simulink model "ILC"  (R2015a)
settings: Solver=ode45  StartTime=0.0  StopTime=7  RelTol=1e-3
undefined symbols (not defined in the file or in its folder): sample_time
libraries: dspadpt3 x7
settings Model: CovSFcnEnable=off  Creator=paulghanem  LastModifiedBy=User
settings DebuggingCC: SolverPrmCheckMsg=warning

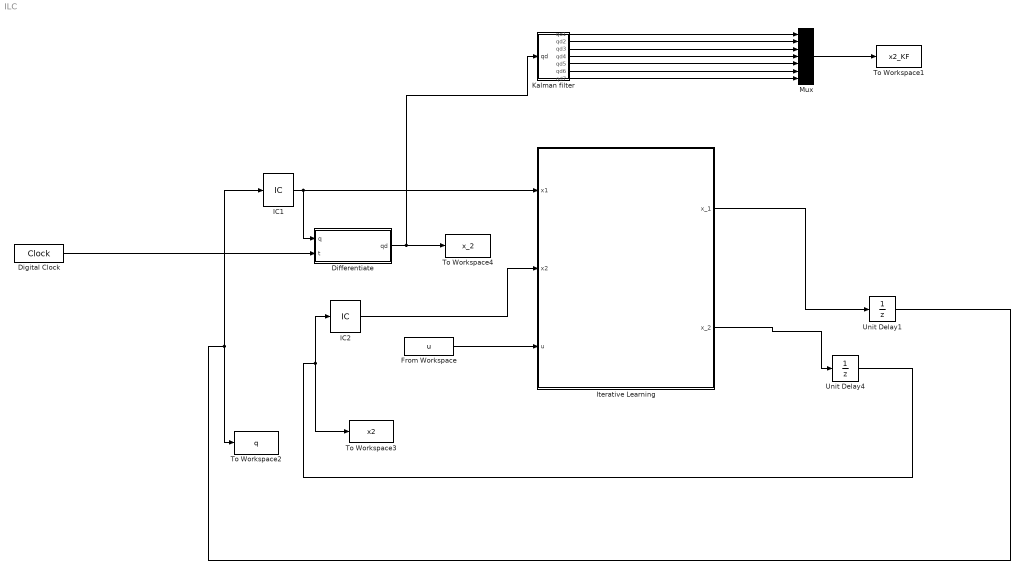
== system ILC ==
  Differentiate : Subsystem
  Digital Clock : DigitalClock  SampleTime=sample_time
  From Workspace : FromWorkspace  VariableName=u  SampleTime=sample_time
  IC1 : InitialCondition  Value=[-0.11060;-2;-0.19200;3.1;0.28250;0.09690;-0.27980]
  IC2 : InitialCondition  Value=[0 0 0 0 0 0 0]
  "Iterative Learning " : MATLAB Function  TreatAsAtomicUnit=on
  Kalman filter : Subsystem
  Mux : Mux  Inputs=7
  To Workspace1 : ToWorkspace  VariableName=x2_KF  SaveFormat=Structure With Time  SampleTime=-1
  To Workspace2 : ToWorkspace  VariableName=q  SaveFormat=Structure With Time  SampleTime=-1
  To Workspace3 : ToWorkspace  VariableName=x2  SaveFormat=Structure With Time  SampleTime=-1
  To Workspace4 : ToWorkspace  VariableName=x_2  SaveFormat=Structure With Time  SampleTime=-1
  Unit Delay1 : UnitDelay  SampleTime=sample_time
  Unit Delay4 : UnitDelay  SampleTime=sample_time
  wires:
  IC1/1 -> "Iterative Learning "/1(x1), Differentiate/1(q)
  "Iterative Learning "/1(x_1) -> Unit Delay1/1
  Unit Delay4/1 -> To Workspace3/1, IC2/1
  Unit Delay1/1 -> To Workspace2/1, IC1/1
  Digital Clock/1 -> Differentiate/2(t)
  From Workspace/1 -> "Iterative Learning "/3(u)
  IC2/1 -> "Iterative Learning "/2(x2)
  "Iterative Learning "/2(x_2) -> Unit Delay4/1
  Differentiate/1(qd) -> Kalman filter/1(qd), To Workspace4/1
  Kalman filter/1(qd1) -> Mux/1
  Kalman filter/2(qd2) -> Mux/2
  Kalman filter/3(qd3) -> Mux/3
  Kalman filter/4(qd4) -> Mux/4
  Kalman filter/5(qd5) -> Mux/5
  Kalman filter/6(qd6) -> Mux/6
  Kalman filter/7(qd7) -> Mux/7
  Mux/1 -> To Workspace1/1

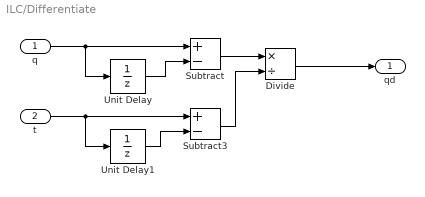
== system ILC/Differentiate ==
  q : Inport
  t : Inport  Port=2
  Divide : Product  Inputs=*/
  Subtract : Sum  Inputs=+-
  Subtract3 : Sum  Inputs=+-
  Unit Delay : UnitDelay  SampleTime=-1
  Unit Delay1 : UnitDelay  SampleTime=-1
  qd : Outport
  wires:
  q/1 -> Subtract/1, Unit Delay/1
  t/1 -> Unit Delay1/1, Subtract3/1
  Unit Delay1/1 -> Subtract3/2
  Unit Delay/1 -> Subtract/2
  Subtract/1 -> Divide/1
  Divide/1 -> qd/1
  Subtract3/1 -> Divide/2

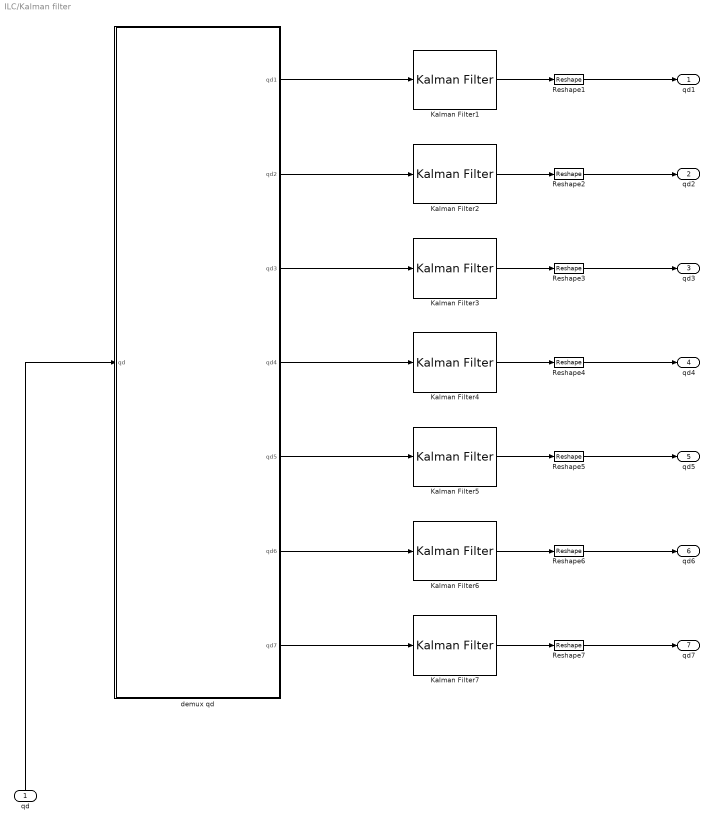
== system ILC/Kalman filter ==
  qd : Inport
  Kalman Filter1 : dspadpt3/Kalman Filter  num_targets=1  sourceEnable=Always  isReset=off  X=[-0.1106; 0]  P=[1e-4 0 ; 0 1]  A=[1 0.002 ; 0 1]  sourceMeasure=Specify via Dialog  H=[1 0]  Q=[0 0.000 ;0.000 0.004]  R=1e-3  isOutputEstMeasure=on  isOutputEstState=off  isOutputEstError=off  isOutputPrdMeasure=off  isOutputPrdState=off  isOutputPrdError=off
  Kalman Filter2 : dspadpt3/Kalman Filter  num_targets=1  sourceEnable=Always  isReset=on  X=[-1.94900000000000; 0]  P=[1e-4 0 ; 0 1]  A=[1 0.002 ; 0 1]  sourceMeasure=Specify via Dialog  H=[1 0]  Q=[0 0; 0 0.004]  R=5e-2  isOutputEstMeasure=on  isOutputEstState=off  isOutputEstError=off  isOutputPrdMeasure=off  isOutputPrdState=off  isOutputPrdError=off
  Kalman Filter3 : dspadpt3/Kalman Filter  num_targets=1  sourceEnable=Always  isReset=on  X=[-0.192000000000000; 0]  P=[1e-4 0 ; 0 1]  A=[1 0.002 ; 0 1]  sourceMeasure=Specify via Dialog  H=[1 0]  Q=[0 0; 0 0.004]  R=1e-3  isOutputEstMeasure=on  isOutputEstState=off  isOutputEstError=off  isOutputPrdMeasure=off  isOutputPrdState=off  isOutputPrdError=off
  Kalman Filter4 : dspadpt3/Kalman Filter  num_targets=1  sourceEnable=Always  isReset=on  X=[3.18400000000000; 0]  P=[1e-4 0 ; 0 1]  A=[1 0.002 ; 0 1]  sourceMeasure=Specify via Dialog  H=[1 0]  Q=[0 0; 0 0.004]  R=1e-3  isOutputEstMeasure=on  isOutputEstState=off  isOutputEstError=off  isOutputPrdMeasure=off  isOutputPrdState=off  isOutputPrdError=off
  Kalman Filter5 : dspadpt3/Kalman Filter  num_targets=1  sourceEnable=Always  isReset=on  X=[0.282500000000000; 0]  P=[1e-4 0 ; 0 1]  A=[1 0.002 ; 0 1]  sourceMeasure=Specify via Dialog  H=[1 0]  Q=[0 0; 0 0.004]  R=1e-6  isOutputEstMeasure=on  isOutputEstState=off  isOutputEstError=off  isOutputPrdMeasure=off  isOutputPrdState=off  isOutputPrdError=off
  Kalman Filter6 : dspadpt3/Kalman Filter  num_targets=1  sourceEnable=Always  isReset=on  X=[0.0969000000000000; 0]  P=[1e-4 0 ; 0 1]  A=[1 0.002 ; 0 1]  sourceMeasure=Specify via Dialog  H=[1 0]  Q=[0 0; 0 0.004]  R=1e-6  isOutputEstMeasure=on  isOutputEstState=off  isOutputEstError=off  isOutputPrdMeasure=off  isOutputPrdState=off  isOutputPrdError=off
  Kalman Filter7 : dspadpt3/Kalman Filter  num_targets=1  sourceEnable=Always  isReset=on  X=[-0.279800000000000; 0]  P=[1e-4 0 ; 0 1]  A=[1 0.002 ; 0 1]  sourceMeasure=Specify via Dialog  H=[1 0]  Q=[0 0; 0 0.004]  R=1e-6  isOutputEstMeasure=on  isOutputEstState=off  isOutputEstError=off  isOutputPrdMeasure=off  isOutputPrdState=off  isOutputPrdError=off
  Reshape{1..7} (7 alike) : Reshape
  demux qd : Subsystem
  qd1 : Outport
  qd2 : Outport  Port=2
  qd3 : Outport  Port=3
  qd4 : Outport  Port=4
  qd5 : Outport  Port=5
  qd6 : Outport  Port=6
  qd7 : Outport  Port=7
  wires:
  Reshape7/1 -> qd7/1
  Kalman Filter7/1 -> Reshape7/1
  qd/1 -> demux qd/1(qd)
  demux qd/7(qd7) -> Kalman Filter7/1
  demux qd/4(qd4) -> Kalman Filter4/1
  Kalman Filter5/1 -> Reshape5/1
  Reshape5/1 -> qd5/1
  demux qd/5(qd5) -> Kalman Filter5/1
  demux qd/2(qd2) -> Kalman Filter2/1
  demux qd/3(qd3) -> Kalman Filter3/1
  Kalman Filter3/1 -> Reshape3/1
  Kalman Filter2/1 -> Reshape2/1
  Reshape3/1 -> qd3/1
  Reshape2/1 -> qd2/1
  demux qd/6(qd6) -> Kalman Filter6/1
  Reshape6/1 -> qd6/1
  Kalman Filter6/1 -> Reshape6/1
  Kalman Filter4/1 -> Reshape4/1
  Reshape4/1 -> qd4/1
  Reshape1/1 -> qd1/1
  Kalman Filter1/1 -> Reshape1/1
  demux qd/1(qd1) -> Kalman Filter1/1

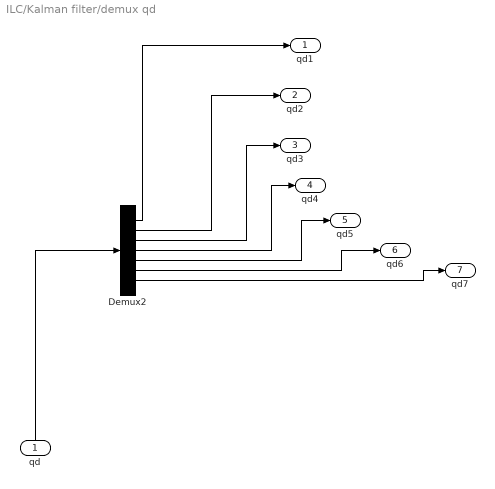
== system ILC/Kalman filter/demux qd ==
  qd : Inport
  Demux2 : Demux  Outputs=7
  qd1 : Outport
  qd2 : Outport  Port=2
  qd3 : Outport  Port=3
  qd4 : Outport  Port=4
  qd5 : Outport  Port=5
  qd6 : Outport  Port=6
  qd7 : Outport  Port=7
  wires:
  qd/1 -> Demux2/1
  Demux2/1 -> qd1/1
  Demux2/2 -> qd2/1
  Demux2/3 -> qd3/1
  Demux2/4 -> qd4/1
  Demux2/5 -> qd5/1
  Demux2/6 -> qd6/1
  Demux2/7 -> qd7/1

== matlab function ILC/Iterative Learning  ==
  data: x1 input; x2 input; u input; x_1 output; x_2 output
function [x_1,x_2]  = fcn(x1,x2,u)
%#codegen
Ts=0.002;
sig = 1e-3;

F1 =  diag([0.20519,0.094428,0.094428,0.03,0.001,0.001,0.0003]);

   C= [zeros(7,7),eye(7)];
 
 
 x11 = x1 + sig*(0.5 - rand(7,1));
 
 
 
 
 



   
    
    
    ff = G(x11);   
    
    
    
    %not to be used in real time
    U=u+ff;
    
    x_1 =  x2*Ts + x11;
    x_2 = (-inv(D(x1)+F1)*(G(x1) + bq(x2)) + inv(D(x1)+F1)*U)*Ts + x2;
     B= [zeros(7,7);inv(D(x1)+F1)];
     x_2(5:7)=zeros(3,1);
     
     
    
end 
function G=G(q)


DH_a = [0 0 0.045 -0.045 0 0 0];
    DH_d = [0 0 .55 0 0.45 0 0.061];
    DH_alpha = [-pi/2 pi/2 -pi/2 pi/2 -pi/2 pi/2 0];

    m = [10.7676 3.87 1.8022 2.4 0.1237 0.4979886 0.07548270];
    
     
    com= zeros(3,7);
    
   com(:,1) = [-0.00443422;0.12189039;-0.00066489];
    com(:,2) = [-0.00236983;0.03105614;0.01542114 ];
    com(:,3) = [-0.03825858;0.20750770;0.00003309];
    com(:,4) = [0.00498512;-0.00022942;0.13271662 ];
    com(:,5) = [0.00008921;0.00511217;0.00435824];
    com(:,6) = [-0.00012262;-0.01703194;0.02468336];
    com(:,7) = [-0.00007974;0.00016313;-0.00323552 ];
     
     % hand_mass =1.385;
      %  DH_d(7) =DH_d(7)+ .0953; % Adding the distance to the hand frame for the Schunk Gripper
       % com(:,7) =(com(:,7).*hand_mass+com(:,7).*m(7))/(hand_mass+m(7)); % Finding the combined center of mass
        %m(7) =m(7)+hand_mass;  
        
    I=zeros(3,3,7);
    T=zeros(4,4,7);
     I(:,:,1) = [0.29486350,-0.00795023,-0.00009311;
                 -0.00795023,0.11350017,-0.00018711;
                -0.00009311,-0.00018711,0.25065343];
    I(:,:,2) =[0.02606840,-0.00001346,-0.00011701;
               -0.00001346,0.01472202,0.00003659;
              -0.00011701,0.00003659,0.01934814];
    I(:,:,3) = [0.13671601,-0.01680434, 0.00000510;
               -0.01680434,0.00588354,-0.00000530;
                0.00000510,-0.00000530,0.13951371];
    I(:,:,4) = [ 0.05719268,0.00001467,0.00008193;
                 0.00001467,0.05716470,-0.00009417;
                 0.00008193,-0.00009417,0.00300441] ;
    I(:,:,5) =[0.00005587,0.00000026,.00000000;
               0.00000026,0.00007817,-0.00000083;
               0.00000000,-0.00000083,0.00006594];
    I(:,:,6) = [0.00093106,0.00000148,-0.00000201;
                0.00000148, 0.00049833,-0.00022162;
               -0.00000201,-0.00022162,0.00057483];
    I(:,:,7) = [0.003167342, 0,0;       % Approximate Inertia Tensor for Schunk Gripper
                0,0.001128942,0;
                 0,0,0.00258007;];  
            
             
for j=1:7,
        a = DH_a(j);
        d = DH_d(j);
        alpha = DH_alpha(j);
        T(:,:,j) = getTransformDH(a, d, alpha, q(j));
end 


comstar=zeros(4,7);

   
    comstar(:,1) = [com(:,1);1];
    comstar(:,2) = [com(:,2);1];
    comstar(:,3) = [com(:,3);1];
    comstar(:,4) = [com(:,4);1];
    comstar(:,5) = [com(:,5);1];
    comstar(:,6) = [com(:,6);1];
    comstar(:,7) = [com(:,7);1];
    
    Q=zeros(4,4);
    
    Q=[0,-1,0,0;
     1,0,0,0;
     0,0,0,0;
     0,0,0,0];
   
 gravity=[0,0,-9.81,0];
 G=zeros(7,1);
   G(1)= -m(1)*gravity*Q*T(:,:,1)*comstar(:,1)-m(2)*gravity*Q*T(:,:,1)*T(:,:,2)*comstar(:,2)-m(3)*gravity*Q*T(:,:,1)*T(:,:,2)*T(:,:,3)*comstar(:,3)-m(4)*gravity*Q*T(:,:,1)*T(:,:,2)*T(:,:,3)*T(:,:,4)*comstar(:,4)-m(5)*gravity*Q*T(:,:,1)*T(:,:,2)*T(:,:,3)*T(:,:,4)*T(:,:,5)*comstar(:,5)-m(6)*gravity*Q*T(:,:,1)*T(:,:,2)*T(:,:,3)*T(:,:,4)*T(:,:,5)*T(:,:,6)*comstar(:,6)-m(7)*gravity*Q*T(:,:,1)*T(:,:,2)*T(:,:,3)*T(:,:,4)*T(:,:,5)*T(:,:,6)*T(:,:,7)*comstar(:,7);   
   G(2)= -m(2)*gravity*T(:,:,1)*Q*T(:,:,2)*comstar(:,2)-m(3)*gravity*T(:,:,1)*Q*T(:,:,2)*T(:,:,3)*comstar(:,3)-m(4)*gravity*T(:,:,1)*Q*T(:,:,2)*T(:,:,3)*T(:,:,4)*comstar(:,4)-m(5)*gravity*T(:,:,1)*Q*T(:,:,2)*T(:,:,3)*T(:,:,4)*T(:,:,5)*comstar(:,5)-m(6)*gravity*T(:,:,1)*Q*T(:,:,2)*T(:,:,3)*T(:,:,4)*T(:,:,5)*T(:,:,6)*comstar(:,6)-m(7)*gravity*T(:,:,1)*Q*T(:,:,2)*T(:,:,3)*T(:,:,4)*T(:,:,5)*T(:,:,6)*T(:,:,7)*comstar(:,7);
   G(3)= -m(3)*gravity*T(:,:,1)*T(:,:,2)*Q*T(:,:,3)*comstar(:,3)-m(4)*gravity*T(:,:,1)*T(:,:,2)*Q*T(:,:,3)*T(:,:,4)*comstar(:,4)-m(5)*gravity*T(:,:,1)*T(:,:,2)*Q*T(:,:,3)*T(:,:,4)*T(:,:,5)*comstar(:,5)-m(6)*gravity*T(:,:,1)*T(:,:,2)*Q*T(:,:,3)*T(:,:,4)*T(:,:,5)*T(:,:,6)*comstar(:,6)-m(7)*gravity*T(:,:,1)*T(:,:,2)*Q*T(:,:,3)*T(:,:,4)*T(:,:,5)*T(:,:,6)*T(:,:,7)*comstar(:,7);
   G(4)= -m(4)*gravity*T(:,:,1)*T(:,:,2)*T(:,:,3)*Q*T(:,:,4)*comstar(:,4)-m(5)*gravity*T(:,:,1)*T(:,:,2)*T(:,:,3)*Q*T(:,:,4)*T(:,:,5)*comstar(:,5)-m(6)*gravity*T(:,:,1)*T(:,:,2)*T(:,:,3)*Q*T(:,:,4)*T(:,:,5)*T(:,:,6)*comstar(:,6)-m(7)*gravity*T(:,:,1)*T(:,:,2)*T(:,:,3)*Q*T(:,:,4)*T(:,:,5)*T(:,:,6)*T(:,:,7)*comstar(:,7);
   G(5)= -m(5)*gravity*T(:,:,1)*T(:,:,2)*T(:,:,3)*T(:,:,4)*Q*T(:,:,5)*comstar(:,5)-m(6)*gravity*T(:,:,1)*T(:,:,2)*T(:,:,3)*T(:,:,4)*Q*T(:,:,5)*T(:,:,6)*comstar(:,6)-m(7)*gravity*T(:,:,1)*T(:,:,2)*T(:,:,3)*T(:,:,4)*Q*T(:,:,5)*T(:,:,6)*T(:,:,7)*comstar(:,7);
   G(6)= -m(6)*gravity*T(:,:,1)*T(:,:,2)*T(:,:,3)*T(:,:,4)*T(:,:,5)*Q*T(:,:,6)*comstar(:,6)-m(7)*gravity*T(:,:,1)*T(:,:,2)*T(:,:,3)*T(:,:,4)*T(:,:,5)*Q*T(:,:,6)*T(:,:,7)*comstar(:,7);
   G(7)= -m(7)*gravity*T(:,:,1)*T(:,:,2)*T(:,:,3)*T(:,:,4)*T(:,:,5)*T(:,:,6)*Q*T(:,:,7)*comstar(:,7);
    
end 
    function T = getTransformDH(a,d,alpha,q)
    ct = cos(q);
    st = sin(q);
    cb = cos(alpha);
    sb = sin(alpha);
    
    T = [ ct, -st*cb,  st*sb, a*ct;
          st,  ct*cb, -ct*sb, a*st;
          0, sb, cb, d;
          0, 0, 0, 1 ];            
 end       
function bq = bq(qd)
 
 
 
s=20;
bc = [2.516; 2.581; 2.038; 0.956; 0.323; 0.315; 0.066];
B =  [1.142; 0.946; 0.309; 0.255; 0.025; 0.039; 0.004];
 
bq = bc.*atan(s*qd)*2/pi+B.*qd;
end 

function D =D(q);
DH_a = [0 0 0.045 -0.045 0 0 0];
    DH_d = [0 0 .55 0 0.45 0 0.061];
    DH_alpha = [-pi/2 pi/2 -pi/2 pi/2 -pi/2 pi/2 0];

    m = [10.7676 3.87 1.8022 2.4 0.1237 0.4979886 0.07548270];
    
     
    com= zeros(3,7);
    
   com(:,1) = [-0.00443422;0.12189039;-0.00066489];
    com(:,2) = [-0.00236983;0.03105614;0.01542114 ];
    com(:,3) = [-0.03825858;0.20750770;0.00003309];
    com(:,4) = [0.00498512;-0.00022942;0.13271662 ];
    com(:,5) = [0.00008921;0.00511217;0.00435824];
    com(:,6) = [-0.00012262;-0.01703194;0.02468336];
    com(:,7) = [-0.00007974;0.00016313;-0.00323552 ];
     
       
        
    I=zeros(3,3,7);
    T=zeros(4,4,7);
     I(:,:,1) = [0.29486350,-0.00795023,-0.00009311;
                 -0.00795023,0.11350017,-0.00018711;
                -0.00009311,-0.00018711,0.25065343];
    I(:,:,2) =[0.02606840,-0.00001346,-0.00011701;
               -0.00001346,0.01472202,0.00003659;
              -0.00011701,0.00003659,0.01934814];
    I(:,:,3) = [0.13671601,-0.01680434, 0.00000510;
               -0.01680434,0.00588354,-0.00000530;
                0.00000510,-0.00000530,0.13951371];
    I(:,:,4) = [ 0.05719268,0.00001467,0.00008193;
                 0.00001467,0.05716470,-0.00009417;
                 0.00008193,-0.00009417,0.00300441] ;
    I(:,:,5) =[0.00005587,0.00000026,.00000000;
               0.00000026,0.00007817,-0.00000083;
               0.00000000,-0.00000083,0.00006594];
    I(:,:,6) = [0.00093106,0.00000148,-0.00000201;
                0.00000148, 0.00049833,-0.00022162;
               -0.00000201,-0.00022162,0.00057483];
    I(:,:,7) = [0.003167342, 0,0;       % Approximate Inertia Tensor for Schunk Gripper
                0,0.001128942,0;
                 0,0,0.00258007;];  
            
             
             
for j=1:7,
        a = DH_a(j);
        d = DH_d(j);
        alpha = DH_alpha(j);
        T(:,:,j) = getTransformDH(a, d, alpha, q(j));
end 

comstar=zeros(4,7);

   
    comstar(:,1) = [com(:,1);1];
    comstar(:,2) = [com(:,2);1];
    comstar(:,3) = [com(:,3);1];
    comstar(:,4) = [com(:,4);1];
    comstar(:,5) = [com(:,5);1];
    comstar(:,6) = [com(:,6);1];
    comstar(:,7) = [com(:,7);1];
    
    Q=zeros(4,4);
    
    Q=[0,-1,0,0;
     1,0,0,0;
     0,0,0,0;
     0,0,0,0];
   

   
U=zeros(4,4,7,7);
   
   U(:,:,1,1)= Q*T(:,:,1);
   U(:,:,2,1)= Q*T(:,:,1)*T(:,:,2);
   U(:,:,3,1)= Q*T(:,:,1)*T(:,:,2)*T(:,:,3);
   U(:,:,4,1)= Q*T(:,:,1)*T(:,:,2)*T(:,:,3)*T(:,:,4);
   U(:,:,5,1)= Q*T(:,:,1)*T(:,:,2)*T(:,:,3)*T(:,:,4)*T(:,:,5);
   U(:,:,6,1)= Q*T(:,:,1)*T(:,:,2)*T(:,:,3)*T(:,:,4)*T(:,:,5)*T(:,:,6);
   U(:,:,7,1)= Q*T(:,:,1)*T(:,:,2)*T(:,:,3)*T(:,:,4)*T(:,:,5)*T(:,:,6)*T(:,:,7);
   
   
   U(:,:,2,2)= T(:,:,1)*Q*T(:,:,2);
   U(:,:,3,2)= T(:,:,1)*Q*T(:,:,2)*T(:,:,3);
   U(:,:,4,2)= T(:,:,1)*Q*T(:,:,2)*T(:,:,3)*T(:,:,4);
   U(:,:,5,2)= T(:,:,1)*Q*T(:,:,2)*T(:,:,3)*T(:,:,4)*T(:,:,5);
   U(:,:,6,2)= T(:,:,1)*Q*T(:,:,2)*T(:,:,3)*T(:,:,4)*T(:,:,5)*T(:,:,6);
   U(:,:,7,2)= T(:,:,1)*Q*T(:,:,2)*T(:,:,3)*T(:,:,4)*T(:,:,5)*T(:,:,6)*T(:,:,7);
   
  
   U(:,:,3,3)= T(:,:,1)*T(:,:,2)*Q*T(:,:,3);
   U(:,:,4,3)= T(:,:,1)*T(:,:,2)*Q*T(:,:,3)*T(:,:,4);
   U(:,:,5,3)= T(:,:,1)*T(:,:,2)*Q*T(:,:,3)*T(:,:,4)*T(:,:,5);
   U(:,:,6,3)= T(:,:,1)*T(:,:,2)*Q*T(:,:,3)*T(:,:,4)*T(:,:,5)*T(:,:,6);
   U(:,:,7,3)= T(:,:,1)*T(:,:,2)*Q*T(:,:,3)*T(:,:,4)*T(:,:,5)*T(:,:,6)*T(:,:,7);
   
   U(:,:,4,4)= T(:,:,1)*T(:,:,2)*T(:,:,3)*Q*T(:,:,4);
   U(:,:,5,4)= T(:,:,1)*T(:,:,2)*T(:,:,3)*Q*T(:,:,4)*T(:,:,5);
   U(:,:,6,4)= T(:,:,1)*T(:,:,2)*T(:,:,3)*Q*T(:,:,4)*T(:,:,5)*T(:,:,6);
   U(:,:,7,4)= T(:,:,1)*T(:,:,2)*T(:,:,3)*Q*T(:,:,4)*T(:,:,5)*T(:,:,6)*T(:,:,7);
   
   U(:,:,5,5)= T(:,:,1)*T(:,:,2)*T(:,:,3)*T(:,:,4)*Q*T(:,:,5);
   U(:,:,6,5)= T(:,:,1)*T(:,:,2)*T(:,:,3)*T(:,:,4)*Q*T(:,:,5)*T(:,:,6);
   U(:,:,7,5)= T(:,:,1)*T(:,:,2)*T(:,:,3)*T(:,:,4)*Q*T(:,:,5)*T(:,:,6)*T(:,:,7);
   
   U(:,:,6,6)= T(:,:,1)*T(:,:,2)*T(:,:,3)*T(:,:,4)*T(:,:,5)*Q*T(:,:,6);
   U(:,:,7,6)= T(:,:,1)*T(:,:,2)*T(:,:,3)*T(:,:,4)*T(:,:,5)*Q*T(:,:,6)*T(:,:,7);
   
   U(:,:,7,7)= T(:,:,1)*T(:,:,2)*T(:,:,3)*T(:,:,4)*T(:,:,5)*T(:,:,6)*Q*T(:,:,7);
   
   
   
  
   J=zeros(4,4,7);
 
   
   J(:,:,1)=[0.5*(-I(1,1,1)+I(2,2,1)+I(3,3,1)), I(1,2,1), I(1,3,1), m(1)*com(1,1);
             I(1,2,1) ,0.5*(I(1,1,1)-I(2,2,1)+I(3,3,1)), I(2,3,1), m(1)*com(2,1);
             I(1,3,1), I(2,3,1), 0.5*(I(1,1,1)+I(2,2,1)-I(3,3,1)), m(1)*com(3,1);
              m(1)*com(1,1), m(1)*com(2,1), m(1)*com(3,1), m(1)];
   
    J(:,:,2)=[0.5*(-I(1,1,2)+I(2,2,2)+I(3,3,2)), I(1,2,2), I(1,3,2), m(2)*com(1,2);
             I(1,2,2) ,0.5*(I(1,1,2)-I(2,2,2)+I(3,3,2)), I(2,3,2), m(2)*com(2,2);
             I(1,3,2), I(2,3,2), 0.5*(I(1,1,2)+I(2,2,2)-I(3,3,2)), m(2)*com(3,2);
              m(2)*com(1,2), m(2)*com(2,2), m(2)*com(3,2), m(2)];
   
          
     J(:,:,3)=[0.5*(-I(1,1,3)+I(2,2,3)+I(3,3,3)), I(1,2,3), I(1,3,3), m(3)*com(1,3);
             I(1,2,3) ,0.5*(I(1,1,3)-I(2,2,3)+I(3,3,3)), I(2,3,3), m(3)*com(2,3);
             I(1,3,3), I(2,3,3), 0.5*(I(1,1,3)+I(2,2,3)-I(3,3,3)), m(3)*com(3,3);
              m(3)*com(1,3), m(3)*com(2,3), m(3)*com(3,3), m(3)];      
   
   
    J(:,:,4)=[0.5*(-I(1,1,4)+I(2,2,4)+I(3,3,4)), I(1,2,4), I(1,3,4), m(4)*com(1,4);
             I(1,2,4) ,0.5*(I(1,1,4)-I(2,2,4)+I(3,3,4)), I(2,3,4), m(4)*com(2,4);
             I(1,3,4), I(2,3,4), 0.5*(I(1,1,4)+I(2,2,4)-I(3,3,4)), m(4)*com(3,4);
              m(4)*com(1,4), m(4)*com(2,4), m(4)*com(3,4), m(4)];
   
   
    J(:,:,5)=[0.5*(-I(1,1,5)+I(2,2,5)+I(3,3,5)), I(1,2,5), I(1,3,5), m(5)*com(1,5);
             I(1,2,5) ,0.5*(I(1,1,5)-I(2,2,5)+I(3,3,5)), I(2,3,5), m(5)*com(2,5);
             I(1,3,5), I(2,3,5), 0.5*(I(1,1,5)+I(2,2,5)-I(3,3,5)), m(5)*com(3,5);
              m(5)*com(1,5), m(5)*com(2,5), m(5)*com(3,5), m(5)];
   
   
    J(:,:,6)=[0.5*(-I(1,1,6)+I(2,2,6)+I(3,3,6)), I(1,2,6), I(1,3,6), m(6)*com(1,6);
             I(1,2,6) ,0.5*(I(1,1,6)-I(2,2,6)+I(3,3,6)), I(2,3,6), m(6)*com(2,6);
             I(1,3,6), I(2,3,6), 0.5*(I(1,1,6)+I(2,2,6)-I(3,3,6)), m(6)*com(3,6);
              m(6)*com(1,6), m(6)*com(2,6), m(6)*com(3,6), m(6)];
   
   
    J(:,:,7)=[0.5*(-I(1,1,7)+I(2,2,7)+I(3,3,7)), I(1,2,7), I(1,3,7), m(7)*com(1,7);
             I(1,2,7) ,0.5*(I(1,1,7)-I(2,2,7)+I(3,3,7)), I(2,3,7), m(7)*com(2,7);
             I(1,3,7), I(2,3,7), 0.5*(I(1,1,7)+I(2,2,7)-I(3,3,7)), m(7)*com(3,7);
              m(7)*com(1,7), m(7)*com(2,7), m(7)*com(3,7), m(7)];
          
          D=zeros(7,7);
   
   
    D(1,1)= trace(U(:,:,1,1)*J(:,:,1)*transpose(U(:,:,1,1))) + trace(U(:,:,2,1)*J(:,:,2)*transpose(U(:,:,2,1))) + trace(U(:,:,3,1)*J(:,:,3)*transpose(U(:,:,3,1))) + trace(U(:,:,4,1)*J(:,:,4)*transpose(U(:,:,4,1))) + trace(U(:,:,5,1)*J(:,:,5)*transpose(U(:,:,5,1))) + trace(U(:,:,6,1)*J(:,:,6)*transpose(U(:,:,6,1))) + trace(U(:,:,7,1)*J(:,:,7)*transpose(U(:,:,7,1))) ;
    D(1,2)= trace(U(:,:,2,2)*J(:,:,2)*transpose(U(:,:,2,1))) + trace(U(:,:,3,2)*J(:,:,3)*transpose(U(:,:,3,1))) + trace(U(:,:,4,2)*J(:,:,4)*transpose(U(:,:,4,1))) +trace(U(:,:,5,2)*J(:,:,5)*transpose(U(:,:,5,1))) + trace(U(:,:,6,2)*J(:,:,6)*transpose(U(:,:,6,1))) + trace(U(:,:,7,2)*J(:,:,7)*transpose(U(:,:,7,1))); 
    D(1,3)= trace(U(:,:,3,3)*J(:,:,3)*transpose(U(:,:,3,1)))+ trace(U(:,:,4,3)*J(:,:,4)*transpose(U(:,:,4,1)))+ trace(U(:,:,5,3)*J(:,:,5)*transpose(U(:,:,5,1)))+ trace(U(:,:,6,3)*J(:,:,6)*transpose(U(:,:,6,1)))+ trace(U(:,:,7,3)*J(:,:,7)*transpose(U(:,:,7,1))); 
    D(1,4)= trace(U(:,:,4,4)*J(:,:,4)*transpose(U(:,:,4,1)))+ trace(U(:,:,5,4)*J(:,:,5)*transpose(U(:,:,5,1)))+ trace(U(:,:,6,4)*J(:,:,6)*transpose(U(:,:,6,1)))+ trace(U(:,:,7,4)*J(:,:,7)*transpose(U(:,:,7,1)));
    D(1,5)= trace(U(:,:,5,5)*J(:,:,5)*transpose(U(:,:,5,1)))+ trace(U(:,:,6,5)*J(:,:,6)*transpose(U(:,:,6,1)))+ trace(U(:,:,7,5)*J(:,:,7)*transpose(U(:,:,7,1)));
    D(1,6)= trace(U(:,:,6,6)*J(:,:,6)*transpose(U(:,:,6,1)))+ trace(U(:,:,7,6)*J(:,:,7)*transpose(U(:,:,7,1)));
    D(1,7)= trace(U(:,:,7,7)*J(:,:,7)*transpose(U(:,:,7,1)));
    
    D(2,1)= trace(U(:,:,2,1)*J(:,:,2)*transpose(U(:,:,2,2)))+ trace(U(:,:,3,1)*J(:,:,3)*transpose(U(:,:,3,2)))+ trace(U(:,:,4,1)*J(:,:,4)*transpose(U(:,:,4,2)))+ trace(U(:,:,5,1)*J(:,:,5)*transpose(U(:,:,5,2)))+ trace(U(:,:,6,1)*J(:,:,6)*transpose(U(:,:,6,2)))+ trace(U(:,:,7,1)*J(:,:,7)*transpose(U(:,:,7,2)));
    D(2,2)= trace(U(:,:,2,2)*J(:,:,2)*transpose(U(:,:,2,2)))+ trace(U(:,:,3,2)*J(:,:,3)*transpose(U(:,:,3,2)))+ trace(U(:,:,4,2)*J(:,:,4)*transpose(U(:,:,4,2)))+ trace(U(:,:,5,2)*J(:,:,5)*transpose(U(:,:,5,2)))+ trace(U(:,:,6,2)*J(:,:,6)*transpose(U(:,:,6,2)))+ trace(U(:,:,7,2)*J(:,:,7)*transpose(U(:,:,7,2)));
    D(2,3)= trace(U(:,:,3,3)*J(:,:,3)*transpose(U(:,:,3,2)))+ trace(U(:,:,4,3)*J(:,:,4)*transpose(U(:,:,4,2)))+ trace(U(:,:,5,3)*J(:,:,5)*transpose(U(:,:,5,2)))+ trace(U(:,:,6,3)*J(:,:,6)*transpose(U(:,:,6,2)))+ trace(U(:,:,7,3)*J(:,:,7)*transpose(U(:,:,7,2))); 
    D(2,4)= trace(U(:,:,4,4)*J(:,:,4)*transpose(U(:,:,4,2)))+ trace(U(:,:,5,4)*J(:,:,5)*transpose(U(:,:,5,2)))+ trace(U(:,:,6,4)*J(:,:,6)*transpose(U(:,:,6,2)))+ trace(U(:,:,7,4)*J(:,:,7)*transpose(U(:,:,7,2))); 
    D(2,5)= trace(U(:,:,5,5)*J(:,:,5)*transpose(U(:,:,5,2)))+ trace(U(:,:,6,5)*J(:,:,6)*transpose(U(:,:,6,2)))+ trace(U(:,:,7,5)*J(:,:,7)*transpose(U(:,:,7,2)));
    D(2,6)= trace(U(:,:,6,6)*J(:,:,6)*transpose(U(:,:,6,2)))+ trace(U(:,:,7,6)*J(:,:,7)*transpose(U(:,:,7,2))); 
    D(2,7)= trace(U(:,:,7,7)*J(:,:,7)*transpose(U(:,:,7,2)));
  
    D(3,1)= trace(U(:,:,3,1)*J(:,:,3)*transpose(U(:,:,3,3)))+ trace(U(:,:,4,1)*J(:,:,4)*transpose(U(:,:,4,3)))+ trace(U(:,:,5,1)*J(:,:,5)*transpose(U(:,:,5,3)))+ trace(U(:,:,6,1)*J(:,:,6)*transpose(U(:,:,6,3)))+ trace(U(:,:,7,1)*J(:,:,7)*transpose(U(:,:,7,3)));
    D(3,2)= trace(U(:,:,3,2)*J(:,:,3)*transpose(U(:,:,3,3)))+ trace(U(:,:,4,2)*J(:,:,4)*transpose(U(:,:,4,3)))+ trace(U(:,:,5,2)*J(:,:,5)*transpose(U(:,:,5,3)))+ trace(U(:,:,6,2)*J(:,:,6)*transpose(U(:,:,6,3)))+ trace(U(:,:,7,2)*J(:,:,7)*transpose(U(:,:,7,3)));
    D(3,3)= trace(U(:,:,3,3)*J(:,:,3)*transpose(U(:,:,3,3)))+ trace(U(:,:,4,3)*J(:,:,4)*transpose(U(:,:,4,3)))+ trace(U(:,:,5,3)*J(:,:,5)*transpose(U(:,:,5,3)))+ trace(U(:,:,6,3)*J(:,:,6)*transpose(U(:,:,6,3)))+ trace(U(:,:,7,3)*J(:,:,7)*transpose(U(:,:,7,3)));
    D(3,4)= trace(U(:,:,4,4)*J(:,:,4)*transpose(U(:,:,4,3)))+ trace(U(:,:,5,4)*J(:,:,5)*transpose(U(:,:,5,3)))+ trace(U(:,:,6,4)*J(:,:,6)*transpose(U(:,:,6,3)))+ trace(U(:,:,7,4)*J(:,:,7)*transpose(U(:,:,7,3)));
    D(3,5)= trace(U(:,:,5,5)*J(:,:,5)*transpose(U(:,:,5,3)))+ trace(U(:,:,6,5)*J(:,:,6)*transpose(U(:,:,6,3)))+ trace(U(:,:,7,5)*J(:,:,7)*transpose(U(:,:,7,3)));
    D(3,6)= trace(U(:,:,6,6)*J(:,:,6)*transpose(U(:,:,6,3)))+ trace(U(:,:,7,6)*J(:,:,7)*transpose(U(:,:,7,3)));
    D(3,7)= trace(U(:,:,7,7)*J(:,:,7)*transpose(U(:,:,7,3)));
     
     
    D(4,1)= trace(U(:,:,4,1)*J(:,:,4)*transpose(U(:,:,4,4)))+ trace(U(:,:,5,1)*J(:,:,5)*transpose(U(:,:,5,4)))+ trace(U(:,:,6,1)*J(:,:,6)*transpose(U(:,:,6,4)))+ trace(U(:,:,7,1)*J(:,:,7)*transpose(U(:,:,7,4))); 
    D(4,2)= trace(U(:,:,4,2)*J(:,:,4)*transpose(U(:,:,4,4)))+ trace(U(:,:,5,2)*J(:,:,5)*transpose(U(:,:,5,4)))+ trace(U(:,:,6,2)*J(:,:,6)*transpose(U(:,:,6,4)))+ trace(U(:,:,7,2)*J(:,:,7)*transpose(U(:,:,7,4))); 
    D(4,3)= trace(U(:,:,4,3)*J(:,:,4)*transpose(U(:,:,4,4)))+ trace(U(:,:,5,3)*J(:,:,5)*transpose(U(:,:,5,4)))+ trace(U(:,:,6,3)*J(:,:,6)*transpose(U(:,:,6,4)))+ trace(U(:,:,7,3)*J(:,:,7)*transpose(U(:,:,7,4)));
    D(4,4)= trace(U(:,:,4,4)*J(:,:,4)*transpose(U(:,:,4,4)))+ trace(U(:,:,5,4)*J(:,:,5)*transpose(U(:,:,5,4)))+ trace(U(:,:,6,4)*J(:,:,6)*transpose(U(:,:,6,4)))+ trace(U(:,:,7,4)*J(:,:,7)*transpose(U(:,:,7,4)));
    D(4,5)= trace(U(:,:,5,5)*J(:,:,5)*transpose(U(:,:,5,4)))+ trace(U(:,:,6,5)*J(:,:,6)*transpose(U(:,:,6,4)))+ trace(U(:,:,7,5)*J(:,:,7)*transpose(U(:,:,7,4)));
    D(4,6)= trace(U(:,:,6,6)*J(:,:,6)*transpose(U(:,:,6,4)))+ trace(U(:,:,7,6)*J(:,:,7)*transpose(U(:,:,7,4))); 
    D(4,7)= trace(U(:,:,7,7)*J(:,:,7)*transpose(U(:,:,7,4)));
    
    D(5,1)= trace(U(:,:,5,1)*J(:,:,5)*transpose(U(:,:,5,5)))+ trace(U(:,:,6,1)*J(:,:,6)*transpose(U(:,:,6,5)))+ trace(U(:,:,7,1)*J(:,:,7)*transpose(U(:,:,7,5)));
    D(5,2)= trace(U(:,:,5,2)*J(:,:,5)*transpose(U(:,:,5,5)))+ trace(U(:,:,6,2)*J(:,:,6)*transpose(U(:,:,6,5)))+ trace(U(:,:,7,2)*J(:,:,7)*transpose(U(:,:,7,5)));
    D(5,3)= trace(U(:,:,5,3)*J(:,:,5)*transpose(U(:,:,5,5)))+ trace(U(:,:,6,3)*J(:,:,6)*transpose(U(:,:,6,5)))+ trace(U(:,:,7,3)*J(:,:,7)*transpose(U(:,:,7,5))); 
    D(5,4)= trace(U(:,:,5,4)*J(:,:,5)*transpose(U(:,:,5,5)))+ trace(U(:,:,6,4)*J(:,:,6)*transpose(U(:,:,6,5)))+ trace(U(:,:,7,4)*J(:,:,7)*transpose(U(:,:,7,5))); 
    D(5,5)= trace(U(:,:,5,5)*J(:,:,5)*transpose(U(:,:,5,5)))+ trace(U(:,:,6,5)*J(:,:,6)*transpose(U(:,:,6,5)))+ trace(U(:,:,7,5)*J(:,:,7)*transpose(U(:,:,7,5)));
    D(5,6)= trace(U(:,:,6,6)*J(:,:,6)*transpose(U(:,:,6,5)))+ trace(U(:,:,7,6)*J(:,:,7)*transpose(U(:,:,7,5))); 
    D(5,7)= trace(U(:,:,7,7)*J(:,:,7)*transpose(U(:,:,7,5)));
    
    D(6,1)= trace(U(:,:,6,1)*J(:,:,6)*transpose(U(:,:,6,6)))+ trace(U(:,:,7,1)*J(:,:,7)*transpose(U(:,:,7,6)));
    D(6,2)= trace(U(:,:,6,2)*J(:,:,6)*transpose(U(:,:,6,6)))+ trace(U(:,:,7,2)*J(:,:,7)*transpose(U(:,:,7,6)));
    D(6,3)= trace(U(:,:,6,3)*J(:,:,6)*transpose(U(:,:,6,6)))+ trace(U(:,:,7,3)*J(:,:,7)*transpose(U(:,:,7,6))); 
    D(6,4)= trace(U(:,:,6,4)*J(:,:,6)*transpose(U(:,:,6,6)))+ trace(U(:,:,7,4)*J(:,:,7)*transpose(U(:,:,7,6))); 
    D(6,5)= trace(U(:,:,6,5)*J(:,:,6)*transpose(U(:,:,6,6)))+ trace(U(:,:,7,5)*J(:,:,7)*transpose(U(:,:,7,6))); 
    D(6,6)= trace(U(:,:,6,6)*J(:,:,6)*transpose(U(:,:,6,6)))+ trace(U(:,:,7,6)*J(:,:,7)*transpose(U(:,:,7,6))); 
    D(6,7)= trace(U(:,:,7,7)*J(:,:,7)*transpose(U(:,:,7,6)));
    
    D(7,1)= trace(U(:,:,7,1)*J(:,:,7)*transpose(U(:,:,7,7)));
    D(7,2)= trace(U(:,:,7,2)*J(:,:,7)*transpose(U(:,:,7,7)));
    D(7,3)= trace(U(:,:,7,3)*J(:,:,7)*transpose(U(:,:,7,7)));
    D(7,4)= trace(U(:,:,7,4)*J(:,:,7)*transpose(U(:,:,7,7)));
    D(7,5)= trace(U(:,:,7,5)*J(:,:,7)*transpose(U(:,:,7,7)));
    D(7,6)= trace(U(:,:,7,6)*J(:,:,7)*transpose(U(:,:,7,7)));
    D(7,7)= trace(U(:,:,7,7)*J(:,:,7)*transpose(U(:,:,7,7)));
end
